simulink model "decoupling_simulation"  (R2014a)
settings: Solver=ode45  StartTime=0.0  StopTime=1000  RelTol=1e-3
libraries: simulink x3
settings Model: Creator=38128  LastModifiedBy=38128

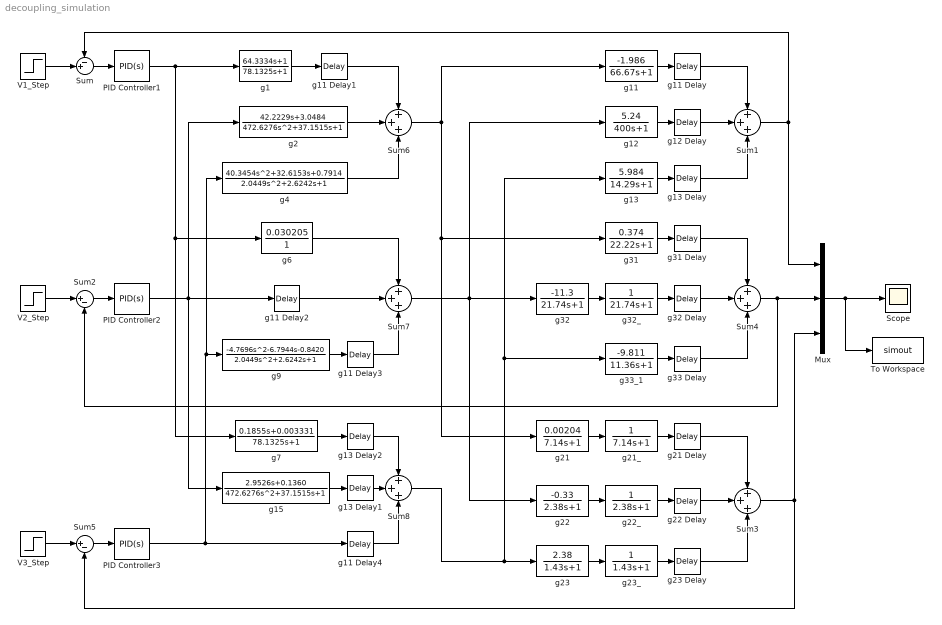
== system decoupling_simulation ==
  Mux : Mux  Inputs=3
  PID Controller1 : simulink/Continuous/PID Controller  Controller=PID  TimeDomain=Continuous-time  SampleTime=1  IntegratorMethod=Forward Euler  FilterMethod=Forward Euler  Form=Parallel  P=-1.9309  I=-0.0247  D=0  N=100  InitialConditionSource=internal  InitialConditionForIntegrator=0  InitialConditionForFilter=0  ExternalReset=none  LimitOutput=off  UpperSaturationLimit=inf  LowerSaturationLimit=-inf  LinearizeAsGain=on  AntiWindupMode=none  Kb=1  TrackingMode=off  Kt=1  PParamMin=[]  PParamMax=[]  IParamMin=[]  IParamMax=[]  DParamMin=[]  DParamMax=[]  NParamMin=[]  NParamMax=[]  KbParamMin=[]  KbParamMax=[]  KtParamMin=[]  KtParamMax=[]  POutMin=[]  POutMax=[]  IOutMin=[]  IOutMax=[]  DOutMin=[]  DOutMax=[]  NOutMin=[]  NOutMax=[]  KbOutMin=[]  KbOutMax=[]  KtOutMin=[]  KtOutMax=[]  IntegratorOutMin=[]  IntegratorOutMax=[]  FilterOutMin=[]  FilterOutMax=[]  SumOutMin=[]  SumOutMax=[]  SumI1OutMin=[]  SumI1OutMax=[]  SumI2OutMin=[]  SumI2OutMax=[]  SumI3OutMin=[]  SumI3OutMax=[]  SumDOutMin=[]  SumDOutMax=[]  SaturationOutMin=[]  SaturationOutMax=[]  IntegratorContinuousStateAttributes=''  IntegratorStateMustResolveToSignalObject=off  IntegratorRTWStateStorageClass=Auto  FilterContinuousStateAttributes=''  FilterStateMustResolveToSignalObject=off  FilterRTWStateStorageClass=Auto
  PID Controller2 : simulink/Continuous/PID Controller  Controller=PID  TimeDomain=Continuous-time  SampleTime=1  IntegratorMethod=Forward Euler  FilterMethod=Forward Euler  Form=Parallel  P=-0.3503  I=-0.0094  D=-1  N=100  InitialConditionSource=internal  InitialConditionForIntegrator=0  InitialConditionForFilter=0  ExternalReset=none  LimitOutput=off  UpperSaturationLimit=inf  LowerSaturationLimit=-inf  LinearizeAsGain=on  AntiWindupMode=none  Kb=1  TrackingMode=off  Kt=1  PParamMin=[]  PParamMax=[]  IParamMin=[]  IParamMax=[]  DParamMin=[]  DParamMax=[]  NParamMin=[]  NParamMax=[]  KbParamMin=[]  KbParamMax=[]  KtParamMin=[]  KtParamMax=[]  POutMin=[]  POutMax=[]  IOutMin=[]  IOutMax=[]  DOutMin=[]  DOutMax=[]  NOutMin=[]  NOutMax=[]  KbOutMin=[]  KbOutMax=[]  KtOutMin=[]  KtOutMax=[]  IntegratorOutMin=[]  IntegratorOutMax=[]  FilterOutMin=[]  FilterOutMax=[]  SumOutMin=[]  SumOutMax=[]  SumI1OutMin=[]  SumI1OutMax=[]  SumI2OutMin=[]  SumI2OutMax=[]  SumI3OutMin=[]  SumI3OutMax=[]  SumDOutMin=[]  SumDOutMax=[]  SaturationOutMin=[]  SaturationOutMax=[]  IntegratorContinuousStateAttributes=''  IntegratorStateMustResolveToSignalObject=off  IntegratorRTWStateStorageClass=Auto  FilterContinuousStateAttributes=''  FilterStateMustResolveToSignalObject=off  FilterRTWStateStorageClass=Auto
  PID Controller3 : simulink/Continuous/PID Controller  Controller=PID  TimeDomain=Continuous-time  SampleTime=1  IntegratorMethod=Forward Euler  FilterMethod=Forward Euler  Form=Parallel  P=0.3034  I=0.1156  D=0.2364  N=100  InitialConditionSource=internal  InitialConditionForIntegrator=0  InitialConditionForFilter=0  ExternalReset=none  LimitOutput=off  UpperSaturationLimit=inf  LowerSaturationLimit=-inf  LinearizeAsGain=on  AntiWindupMode=none  Kb=1  TrackingMode=off  Kt=1  PParamMin=[]  PParamMax=[]  IParamMin=[]  IParamMax=[]  DParamMin=[]  DParamMax=[]  NParamMin=[]  NParamMax=[]  KbParamMin=[]  KbParamMax=[]  KtParamMin=[]  KtParamMax=[]  POutMin=[]  POutMax=[]  IOutMin=[]  IOutMax=[]  DOutMin=[]  DOutMax=[]  NOutMin=[]  NOutMax=[]  KbOutMin=[]  KbOutMax=[]  KtOutMin=[]  KtOutMax=[]  IntegratorOutMin=[]  IntegratorOutMax=[]  FilterOutMin=[]  FilterOutMax=[]  SumOutMin=[]  SumOutMax=[]  SumI1OutMin=[]  SumI1OutMax=[]  SumI2OutMin=[]  SumI2OutMax=[]  SumI3OutMin=[]  SumI3OutMax=[]  SumDOutMin=[]  SumDOutMax=[]  SaturationOutMin=[]  SaturationOutMax=[]  IntegratorContinuousStateAttributes=''  IntegratorStateMustResolveToSignalObject=off  IntegratorRTWStateStorageClass=Auto  FilterContinuousStateAttributes=''  FilterStateMustResolveToSignalObject=off  FilterRTWStateStorageClass=Auto
  Scope : Scope
  Sum : Sum  Inputs=-+|
  Sum{1,3..4,6..8} (6 alike) : Sum  Inputs=+++
  Sum2 : Sum  Inputs=|+-
  Sum5 : Sum  Inputs=|+-
  To Workspace : ToWorkspace  VariableName=simout  SaveFormat=Timeseries  SampleTime=-1
  V1_Step : Step  SampleTime=0
  V2_Step : Step  Time=250  SampleTime=0
  V3_Step : Step  Time=500  SampleTime=0
  g1 : TransferFcn  Numerator=[64.3334 1]  Denominator=[78.1325 1]
  g11 : TransferFcn  Numerator=[-1.986]  Denominator=[66.67 1]
  g11 Delay : TransportDelay  DelayTime=0.71
  g11 Delay1 : TransportDelay  DelayTime=11.0348
  g11 Delay2 : TransportDelay  DelayTime=1.5926
  g11 Delay3 : TransportDelay  DelayTime=0.55
  g11 Delay4 : TransportDelay  DelayTime=1.3174
  g12 : TransferFcn  Numerator=[5.24]  Denominator=[400 1]
  g12 Delay : TransportDelay  DelayTime=60
  g13 : TransferFcn  Numerator=[5.984]  Denominator=[14.29 1]
  g13 Delay : TransportDelay  DelayTime=2.24
  g13 Delay1 : TransportDelay  DelayTime=1.7933
  g13 Delay2 : TransportDelay  DelayTime=2.9894
  g15 : TransferFcn  Numerator=[2.9526 0.1360]  Denominator=[472.6276 37.1515 1]
  g2 : TransferFcn  Numerator=[42.2229 3.0484]  Denominator=[472.6276 37.1515 1]
  g21 : TransferFcn  Numerator=[0.00204]  Denominator=[7.14 1]
  g21 Delay : TransportDelay  DelayTime=0.59
  g21_ : TransferFcn  Denominator=[7.14 1]
  g22 : TransferFcn  Numerator=[-0.33]  Denominator=[2.38 1]
  g22 Delay : TransportDelay  DelayTime=0.68
  g22_ : TransferFcn  Denominator=[2.38 1]
  g23 : TransferFcn  Numerator=[2.38]  Denominator=[1.43 1]
  g23 Delay : TransportDelay  DelayTime=0.42
  g23_ : TransferFcn  Denominator=[1.43 1]
  g31 : TransferFcn  Numerator=[0.374]  Denominator=[22.22 1]
  g31 Delay : TransportDelay  DelayTime=7.75
  g32 : TransferFcn  Numerator=[-11.3]  Denominator=[21.74 1]
  g32 Delay : TransportDelay  DelayTime=3.79
  g32_ : TransferFcn  Denominator=[21.74 1]
  g33 Delay : TransportDelay  DelayTime=1.59
  g33_1 : TransferFcn  Numerator=[-9.811]  Denominator=[11.36 1]
  g4 : TransferFcn  Numerator=[40.3454 32.6153 0.7914]  Denominator=[2.0449 2.6242 1]
  g6 : TransferFcn  Numerator=[ 0.030205]  Denominator=[1]
  g7 : TransferFcn  Numerator=[0.1855 0.003331]  Denominator=[78.1325 1]
  g9 : TransferFcn  Numerator=[-4.7696 -6.7944 -0.8420]  Denominator=[2.0449 2.6242 1]
  wires:
  Sum/1 -> PID Controller1/1
  Sum5/1 -> PID Controller3/1
  V1_Step/1 -> Sum/2
  Sum2/1 -> PID Controller2/1
  Mux/1 -> Scope/1, To Workspace/1
  g1/1 -> g11 Delay1/1
  g11 Delay1/1 -> Sum6/1
  g2/1 -> Sum6/2
  PID Controller1/1 -> g1/1, g7/1, g6/1
  g6/1 -> Sum7/1
  g11 Delay2/1 -> Sum7/2
  g11 Delay3/1 -> Sum7/3
  g13 Delay2/1 -> Sum8/1
  g13 Delay1/1 -> Sum8/2
  g11 Delay4/1 -> Sum8/3
  g7/1 -> g13 Delay2/1
  PID Controller2/1 -> g11 Delay2/1, g2/1, g15/1
  g9/1 -> g11 Delay3/1
  g15/1 -> g13 Delay1/1
  PID Controller3/1 -> g11 Delay4/1, g9/1, g4/1
  Sum6/1 -> g11/1, g31/1, g21/1
  g11/1 -> g11 Delay/1
  g11 Delay/1 -> Sum1/1
  g12/1 -> g12 Delay/1
  g13/1 -> g13 Delay/1
  g12 Delay/1 -> Sum1/2
  g13 Delay/1 -> Sum1/3
  g21_/1 -> g21 Delay/1
  g21 Delay/1 -> Sum3/1
  g22_/1 -> g22 Delay/1
  g22 Delay/1 -> Sum3/2
  g23 Delay/1 -> Sum3/3
  g21/1 -> g21_/1
  g22/1 -> g22_/1
  g23_/1 -> g23 Delay/1
  g23/1 -> g23_/1
  g31/1 -> g31 Delay/1
  g31 Delay/1 -> Sum4/1
  g32_/1 -> g32 Delay/1
  g32 Delay/1 -> Sum4/2
  g33 Delay/1 -> Sum4/3
  g32/1 -> g32_/1
  g33_1/1 -> g33 Delay/1
  Sum7/1 -> g32/1, g12/1, g22/1
  Sum8/1 -> g23/1, g33_1/1, g13/1
  Sum1/1 -> Sum/1, Mux/1
  Sum4/1 -> Mux/2, Sum2/2
  Sum3/1 -> Sum5/2, Mux/3
  g4/1 -> Sum6/3
  V3_Step/1 -> Sum5/1
  V2_Step/1 -> Sum2/1
